simulink model "stab_model"  (R2023b)
settings: Solver=VariableStepAuto  StartTime=0.0  StopTime=Tmdl  RelTol=1e-3
undefined symbols (not defined in the file): Ad, Bd, C, K, L, T, x_hat_initial, x_initial
settings Model: Creator=deniskirbaba  LastModifiedBy=deniskirbaba

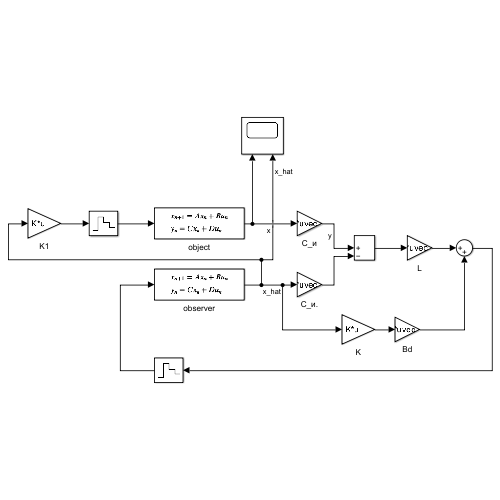
[thumbnail: Simulink's stored preview of the top-level diagram]
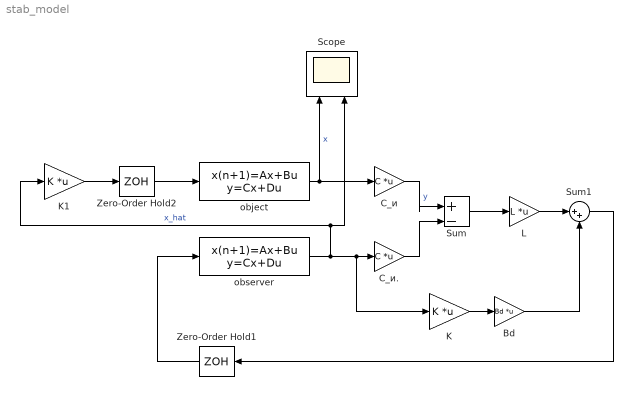
== system stab_model ==
  Bd : Gain  Gain=Bd  Multiplication=Matrix(K*u) (u vector)
  C_и : Gain  Gain=C  Multiplication=Matrix(K*u) (u vector)
  C_и. : Gain  Gain=C  Multiplication=Matrix(K*u) (u vector)
  K : Gain  Gain=K  Multiplication=Matrix(K*u)
  K1 : Gain  Gain=K  Multiplication=Matrix(K*u)
  L : Gain  Gain=L  Multiplication=Matrix(K*u) (u vector)
  Scope : Scope  NumInputPorts=2
  Sum : Sum  Inputs=|+-
  Sum1 : Sum  Inputs=|++
  Zero-Order Hold1 : ZeroOrderHold  SampleTime=T
  Zero-Order Hold2 : ZeroOrderHold  SampleTime=T
  object : DiscreteStateSpace  A=Ad  B=Bd  C=eye(2)  D=[0;0]  InitialCondition=x_initial  SampleTime=-1
  observer : DiscreteStateSpace  A=Ad  B=eye(2)  C=eye(2)  D=[0 0;0 0]  InitialCondition=x_hat_initial  SampleTime=-1
  wires:
  object/1 -> C_и/1, Scope/1  "x"
  C_и/1 -> Sum/1  "y"
  C_и./1 -> Sum/2
  Sum/1 -> L/1
  L/1 -> Sum1/1
  observer/1 -> K1/1, Scope/2, K/1, C_и./1  "x_hat"
  Zero-Order Hold2/1 -> object/1
  K/1 -> Bd/1
  Bd/1 -> Sum1/2
  Sum1/1 -> Zero-Order Hold1/1
  Zero-Order Hold1/1 -> observer/1
  K1/1 -> Zero-Order Hold2/1
